simulink model "ModeloSistema"  (Simulink 9.1)
settings: Solver=ode45  StartTime=0.0  StopTime=20.0  RelTol=1e-3  EnableMultiTasking=on
values from neighbouring files (symbols this model uses):
  a0 = 1    [Aplicacion.m]
  a1 = 2    [Aplicacion.m]
  a2 = 4    [Aplicacion.m]
  a3 = 2    [Aplicacion.m]
  a4 = 2    [Aplicacion.m]
settings Model: SuppressorTable=22 serialization::archive 11 0 6 0 0 0 1 0  Creator=GEO  LastModifiedBy=daniel
settings DataIOCC: LimitDataPoints=on  SignalLoggingSaveFormat=ModelDataLogs
settings DebuggingCC: SaveWithParameterizedLinksMsg=none  SolverPrmCheckMsg=warning  MultiTaskDSMMsg=warning  MultiTaskCondExecSysMsg=none

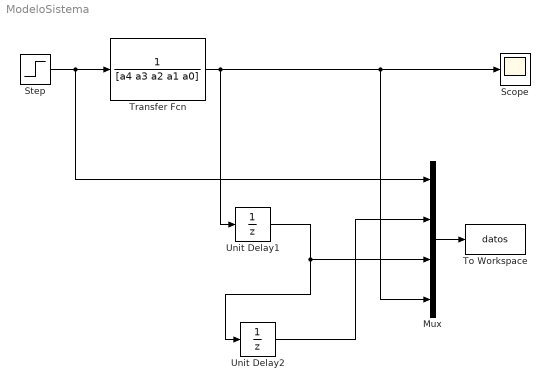
== system ModeloSistema ==
  Mux : Mux
  Scope : Scope
  Step : Step  Time=0.5  SampleTime=0
  To Workspace : ToWorkspace  VariableName=datos  SampleTime=0.1
  Transfer Fcn : TransferFcn  Denominator=[a4 a3 a2 a1 a0]
  Unit Delay1 : UnitDelay  SampleTime=0.1
  Unit Delay2 : UnitDelay  SampleTime=0.1
  wires:
  Step/1 -> Mux/1, Transfer Fcn/1
  Transfer Fcn/1 -> Unit Delay1/1, Scope/1, Mux/4
  Mux/1 -> To Workspace/1
  Unit Delay1/1 -> Unit Delay2/1, Mux/3
  Unit Delay2/1 -> Mux/2
